simulink subsystem "quat_dyn_body"  (R2022a)
settings: Solver=VariableStepAuto  StartTime=0.0  StopTime=10.0  RelTol=1e-3
libraries: matrix_library x1, aerolibutil x1
settings Model: Creator=samuel  LastModifiedBy=samuel

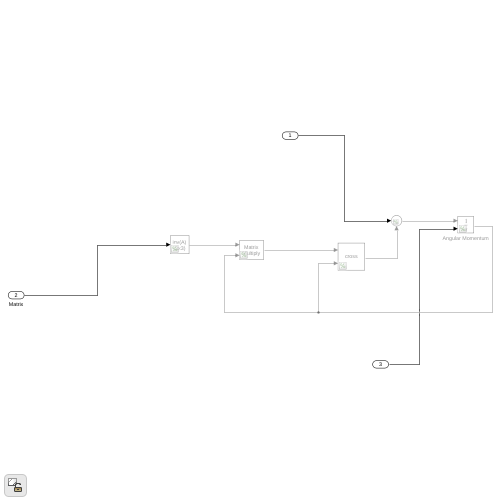
[thumbnail: Simulink's stored preview of the top-level diagram]
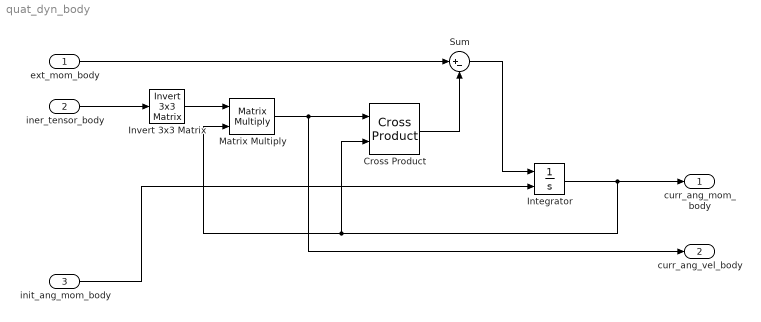
== system quat_dyn_body ==
  ext_mom_body : Inport
  iner_tensor_body : Inport  Port=2
  init_ang_mom_body : Inport  Port=3
  Cross Product : matrix_library/Cross Product
      settings: SourceProductBaseCode=SL
  Integrator : Integrator  InitialConditionSource=external
  Invert 3x3 Matrix : aerolibutil/Invert  3x3 Matrix
  Matrix Multiply : Product  Multiplication=Matrix(*)
  Sum : Sum  Inputs=|+-
  curr_ang_mom_body : Outport
  curr_ang_vel_body : Outport  Port=2
  wires:
  Sum/1 -> Integrator/1
  Matrix Multiply/1 -> Cross Product/1, curr_ang_vel_body/1
  ext_mom_body/1 -> Sum/1
  Integrator/1 -> Cross Product/2, Matrix Multiply/2, curr_ang_mom_body/1
  init_ang_mom_body/1 -> Integrator/2
  iner_tensor_body/1 -> Invert 3x3 Matrix/1
  Cross Product/1 -> Sum/2
  Invert 3x3 Matrix/1 -> Matrix Multiply/1
